simulink model "pwm_rc_opamp_cc_model"  (R2025a)
settings: Solver=ode23tb  StartTime=0.0  StopTime=0.02  MaxStep=1e-6  RelTol=1e-4
model workspace (MAT data in the model file):
  C_FILT = 1e-06
  F_OPAMP = 20000
  I_LIMIT = 3
  K_MOS = 1.2
  K_OPAMP = 300
  PWM_FREQ = 48000
  RLOAD = 1
  R_FILT = 10000
  R_SENSE = 0.1
  TAU_I = 0.0002
  VBOOST = 24
  VDD = 3.3
  VLED = 20
  VTH = 2.2
libraries: simulink x1
settings Model: Creator=banzang  LastModifiedBy=banzang

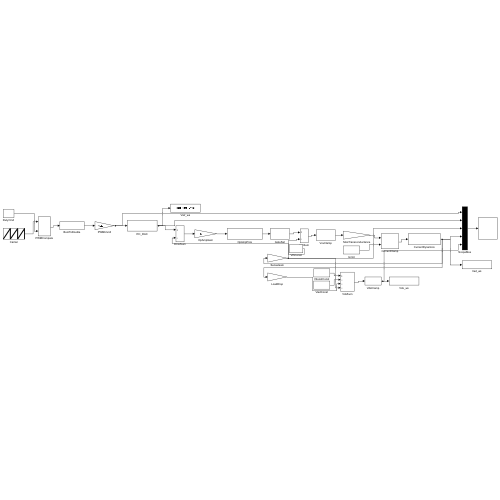
[thumbnail: Simulink's stored preview of the top-level diagram]
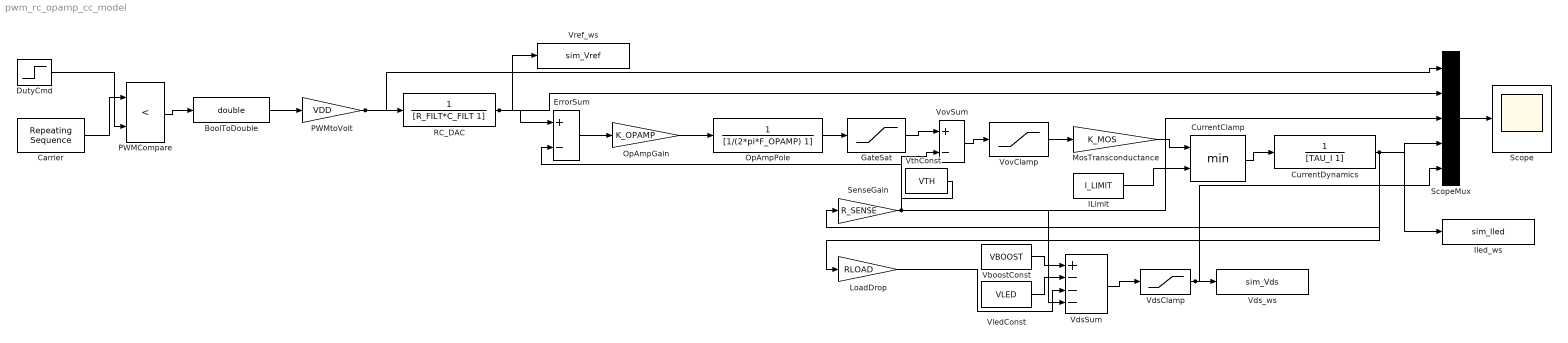
== system pwm_rc_opamp_cc_model ==
  BoolToDouble : DataTypeConversion  OutDataTypeStr=double  SaturateOnIntegerOverflow=off  RndMeth=Floor
  Carrier : simulink/Sources/Repeating Sequence  rep_seq_t=[0 1/PWM_FREQ]  rep_seq_y=[0 1]
  CurrentClamp : MinMax  Inputs=2
  CurrentDynamics : TransferFcn  Numerator=1  Denominator=[TAU_I 1]
  DutyCmd : Step  Time=0.01  Before=0.35  After=0.55  SampleTime=0
  ErrorSum : Sum  Inputs=+-
  GateSat : Saturate  UpperLimit=10  LowerLimit=0
  ILimit : Constant  Value=I_LIMIT
  Iled_ws : ToWorkspace  VariableName=sim_Iled  SaveFormat=Structure With Time  SampleTime=-1
  LoadDrop : Gain  Gain=RLOAD
  MosTransconductance : Gain  Gain=K_MOS
  OpAmpGain : Gain  Gain=K_OPAMP
  OpAmpPole : TransferFcn  Numerator=1  Denominator=[1/(2*pi*F_OPAMP) 1]
  PWMCompare : RelationalOperator  Operator=<  OutDataTypeStr=boolean  RndMeth=Simplest  InputSameDT=off
  PWMtoVolt : Gain  Gain=VDD
  RC_DAC : TransferFcn  Numerator=1  Denominator=[R_FILT*C_FILT 1]
  Scope : Scope
  ScopeMux : Mux  Inputs=5
  SenseGain : Gain  Gain=R_SENSE
  VboostConst : Constant  Value=VBOOST
  VdsClamp : Saturate  UpperLimit=inf  LowerLimit=0
  VdsSum : Sum  Inputs=+---
  Vds_ws : ToWorkspace  VariableName=sim_Vds  SaveFormat=Structure With Time  SampleTime=-1
  VledConst : Constant  Value=VLED
  VovClamp : Saturate  UpperLimit=10  LowerLimit=0
  VovSum : Sum  Inputs=+-
  Vref_ws : ToWorkspace  VariableName=sim_Vref  SaveFormat=Structure With Time  SampleTime=-1
  VthConst : Constant  Value=VTH
  wires:
  DutyCmd/1 -> PWMCompare/2
  Carrier/1 -> PWMCompare/1
  PWMCompare/1 -> BoolToDouble/1
  BoolToDouble/1 -> PWMtoVolt/1
  PWMtoVolt/1 -> RC_DAC/1, ScopeMux/1
  RC_DAC/1 -> ErrorSum/1, Vref_ws/1, ScopeMux/2
  SenseGain/1 -> ErrorSum/2, VdsSum/4, ScopeMux/3
  ErrorSum/1 -> OpAmpGain/1
  OpAmpGain/1 -> OpAmpPole/1
  OpAmpPole/1 -> GateSat/1
  GateSat/1 -> VovSum/1
  VthConst/1 -> VovSum/2
  VovSum/1 -> VovClamp/1
  VovClamp/1 -> MosTransconductance/1
  MosTransconductance/1 -> CurrentClamp/1
  ILimit/1 -> CurrentClamp/2
  CurrentClamp/1 -> CurrentDynamics/1
  CurrentDynamics/1 -> SenseGain/1, LoadDrop/1, Iled_ws/1, ScopeMux/4
  VboostConst/1 -> VdsSum/1
  VledConst/1 -> VdsSum/2
  LoadDrop/1 -> VdsSum/3
  VdsSum/1 -> VdsClamp/1
  VdsClamp/1 -> Vds_ws/1, ScopeMux/5
  ScopeMux/1 -> Scope/1
